simulink model "ThreephaseInverterTrialOut"  (R2016a)
settings: Solver=FixedStepAuto  StartTime=0  StopTime=time  FixedStep=Ts1  RelTol=1  AbsTol=0.1
undefined symbols (not defined in the file or in its folder): f, Ts, Ts1, Vs, Vt
libraries: nesl_utility x12, elec_lib x7, fl_lib x6, pe_lib x6, powerlib_meascontrol x1, powerlib x1
settings Model: Creator=syf  LastModifiedBy=syf

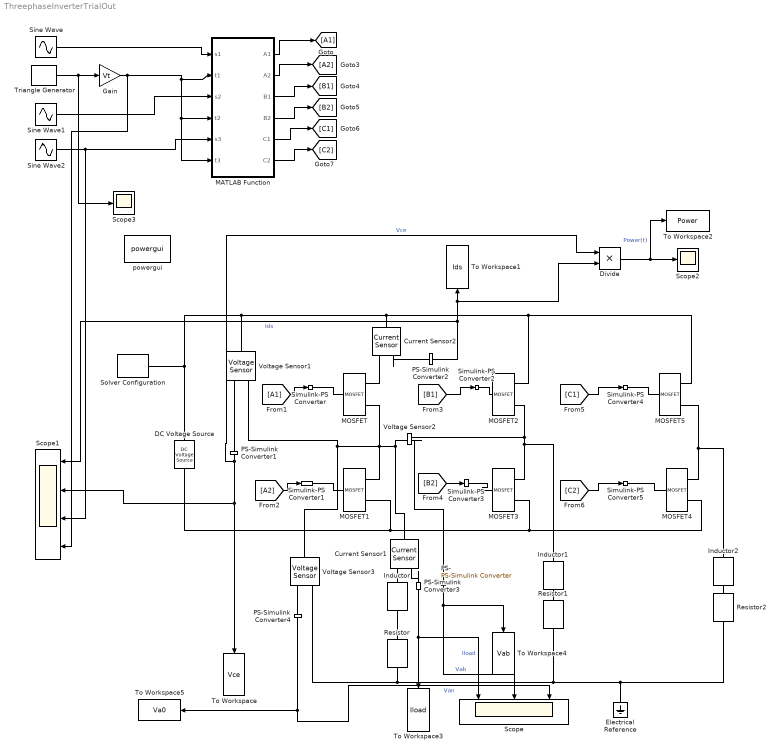
== system ThreephaseInverterTrialOut ==
  Current Sensor1 : fl_lib/Electrical/Electrical Sensors/Current Sensor
  Current Sensor2 : fl_lib/Electrical/Electrical Sensors/Current Sensor
  DC Voltage Source : elec_lib/Additional Components/SPICE-Compatible Components/Sources/DC Voltage Source  DC=650 V
  Divide : Product  Inputs=**
  Electrical Reference : fl_lib/Electrical/Electrical Elements/Electrical Reference
  Gain : Gain  Gain=Vt
  Inductor : elec_lib/Passive Devices/Inductor  l=Ls H  L_tol=20  enable_L_tol=0  tol_distribution=1  nSigma=4  r=0 Ohm  g=1e-9 1/Ohm  initI=0 A  enable_operating_limits=0  operating_limit_action=2  max_working_current=1 A  power_rating=1 W  enable_faults=0  fault_action=1  lambdaPercent=50  k_faulted=0.9999 Ohm  turnsShort=0  openCct=0  groundShort=0  groundShortG=0 1/Ohm  tau_fault=0.001 s  enable_temporal_fault=0  t_fault=1 s  enable_behavioral_fault=0  max_permissible_voltage=100 V  n_fail_on_voltage=1  max_permissible_current=1 A  t_fail_on_current=1 s
  Inductor1 : elec_lib/Passive Devices/Inductor  l=Ls H  L_tol=20  enable_L_tol=0  tol_distribution=1  nSigma=4  r=0 Ohm  g=1e-9 1/Ohm  initI=0 A  enable_operating_limits=0  operating_limit_action=2  max_working_current=1 A  power_rating=1 W  enable_faults=0  fault_action=1  lambdaPercent=50  k_faulted=0.9999 Ohm  turnsShort=0  openCct=0  groundShort=0  groundShortG=0 1/Ohm  tau_fault=0.001 s  enable_temporal_fault=0  t_fault=1 s  enable_behavioral_fault=0  max_permissible_voltage=100 V  n_fail_on_voltage=1  max_permissible_current=1 A  t_fail_on_current=1 s
  Inductor2 : elec_lib/Passive Devices/Inductor  l=Ls H  L_tol=20  enable_L_tol=0  tol_distribution=1  nSigma=4  r=0 Ohm  g=1e-9 1/Ohm  initI=0 A  enable_operating_limits=0  operating_limit_action=2  max_working_current=1 A  power_rating=1 W  enable_faults=0  fault_action=1  lambdaPercent=50  k_faulted=0.9999 Ohm  turnsShort=0  openCct=0  groundShort=0  groundShortG=0 1/Ohm  tau_fault=0.001 s  enable_temporal_fault=0  t_fault=1 s  enable_behavioral_fault=0  max_permissible_voltage=100 V  n_fail_on_voltage=1  max_permissible_current=1 A  t_fail_on_current=1 s
  MATLAB Function : MATLAB Function  TreatAsAtomicUnit=on
  MOSFET{,1..5} (6 alike) : pe_lib/Semiconductors/Fundamental Components/MOSFET  Rds=0.01 Ohm  Goff=1e-6 1/Ohm  Vth=2 V  diode_param=2  diode_Vf=0.8 V  diode_Ron=0.001 Ohm  diode_Goff=1e-5 1/Ohm  diode_C=5e-8 F  diode_iRM=-235 A  diode_iF=300 A  diode_idot=-50 A/us  diode_trr_param=1  diode_trr_factor=3  diode_trr=15 us  diode_Qrr=1.5e+3 s*uA
  "PS- " : nesl_utility/PS-Simulink Converter  PhysicalDomain=network_engine_domain  SubClassName=ps_output  LeftPortType=input  RightPortType=output  PseudoPeriodic=off  Frequencies=[]  Unit=1  AffineConversion=off
  PS-Simulink Converter{1..4} (4 alike) : nesl_utility/PS-Simulink Converter  PhysicalDomain=network_engine_domain  SubClassName=ps_output  LeftPortType=input  RightPortType=output  PseudoPeriodic=off  Frequencies=[]  Unit=1  AffineConversion=off
  Resistor : elec_lib/Passive Devices/Resistor  R=20 Ohm  R_tol=5  enable_R_tol=0  tol_distribution=1  nSigma=4  enable_operating_limits=0  operating_limit_action=2  max_working_voltage=100 V  power_rating=1 W  enable_faults=0  fault_action=1  R_faulted=Inf Ohm  enable_temporal_fault=0  t_fault=1 s  enable_behavioral_fault=0  max_permissible_current=1 A  t_fail_on_current=1 s  noise_mode=0  sample_time=0.001 s  repeatability=1  auto_seed=2843309574  user_seed=0  Tdevice=25 degC  alpha=0.00393 1/K  Tmeas=25 degC  thermal_mass=100 J/K  initial_temperature=25 degC  power_derating_T1=70 degC  power_derating_T2=155 degC  operating_temperature_range_vec=[ -50 150 ] degC
  Resistor1 : elec_lib/Passive Devices/Resistor  R=20 Ohm  R_tol=5  enable_R_tol=0  tol_distribution=1  nSigma=4  enable_operating_limits=0  operating_limit_action=2  max_working_voltage=100 V  power_rating=1 W  enable_faults=0  fault_action=1  R_faulted=Inf Ohm  enable_temporal_fault=0  t_fault=1 s  enable_behavioral_fault=0  max_permissible_current=1 A  t_fail_on_current=1 s  noise_mode=0  sample_time=0.001 s  repeatability=1  auto_seed=1846498393  user_seed=0  Tdevice=25 degC  alpha=0.00393 1/K  Tmeas=25 degC  thermal_mass=100 J/K  initial_temperature=25 degC  power_derating_T1=70 degC  power_derating_T2=155 degC  operating_temperature_range_vec=[ -50 150 ] degC
  Resistor2 : elec_lib/Passive Devices/Resistor  R=20 Ohm  R_tol=5  enable_R_tol=0  tol_distribution=1  nSigma=4  enable_operating_limits=0  operating_limit_action=2  max_working_voltage=100 V  power_rating=1 W  enable_faults=0  fault_action=1  R_faulted=Inf Ohm  enable_temporal_fault=0  t_fault=1 s  enable_behavioral_fault=0  max_permissible_current=1 A  t_fail_on_current=1 s  noise_mode=0  sample_time=0.001 s  repeatability=1  auto_seed=3812947214  user_seed=0  Tdevice=25 degC  alpha=0.00393 1/K  Tmeas=25 degC  thermal_mass=100 J/K  initial_temperature=25 degC  power_derating_T1=70 degC  power_derating_T2=155 degC  operating_temperature_range_vec=[ -50 150 ] degC
  Scope : Scope  NumInputPorts=3
  Scope1 : Scope  NumInputPorts=4
  Scope2 : Scope
  Scope3 : Scope
  Simulink-PS Converter{,1..5} (6 alike) : nesl_utility/Simulink-PS Converter  PhysicalDomain=network_engine_domain  SubClassName=ps_input  LeftPortType=input  RightPortType=output  PseudoPeriodic=off  Frequencies=[]  NoiseDistribution=none  NoiseParameters=[]  Unit=1  AffineConversion=off  InputFiltering=off  SimscapeFilterOrder=1  InputFilterTimeConstant=0.001  UdotUserProvided=1
  Sine Wave : Sin  Amplitude=Vs  Frequency=f*2*pi  SampleTime=0
  Sine Wave1 : Sin  Amplitude=Vs  Frequency=f*2*pi  Phase=2/3*pi  SampleTime=0
  Sine Wave2 : Sin  Amplitude=Vs  Frequency=f*2*pi  Phase=-2/3*pi  SampleTime=0
  Solver Configuration : nesl_utility/Solver Configuration  PhysicalDomain=network_engine_domain  SubClassName=solver  LeftPortType=input  RightPortType=generic  Accelerate=off  Tones=[]  Harmonics=[]  SimulateNoise=off  Profile=off  UseLocalSampling=off  EnableSwitchedLinearOptims=on  FrequencyDomain=off  UseCCode=off  RelTol=0.001  AbsTol=1e-06  MinStep=1e-09  ToWorkspace=off  RevertToSquareIcSolve=off  NumHomotopyIterations=100  PhasorMode=off  PhasorModeNumHarmonics=1  OverrideAbsTol=off  DoDC=off  ResidualTolerance=1e-9  UseLocalSolver=off  LocalSolverChoice=NE_BACKWARD_EULER_ADVANCER  LocalSolverSampleTime=0.001  DoFixedCost=off  MaxNonlinIter=3  MaxModeIter=2  LinearAlgebra=Sparse  DelaysMemoryBudget=1024  AutomaticFiltering=on  FilteringTimeConstant=0.001
  To Workspace : ToWorkspace  VariableName=Vce  SaveFormat=Structure With Time  SampleTime=-1
      settings: Save2DSignal=2-D array (concatenate along first dimension)
  To Workspace1 : ToWorkspace  VariableName=Ids  SaveFormat=Structure With Time  SampleTime=-1
  To Workspace2 : ToWorkspace  VariableName=Power  SampleTime=-1
  To Workspace3 : ToWorkspace  VariableName=Iload  SaveFormat=Structure With Time  SampleTime=-1
      settings: Save2DSignal=2-D array (concatenate along first dimension)
  To Workspace4 : ToWorkspace  VariableName=Vab  SaveFormat=Structure With Time  SampleTime=-1
      settings: Save2DSignal=2-D array (concatenate along first dimension)
  To Workspace5 : ToWorkspace  VariableName=Va0  SaveFormat=Structure With Time  SampleTime=-1
      settings: Save2DSignal=2-D array (concatenate along first dimension)
  Triangle Generator : powerlib_meascontrol/Pulse & Signal Generators/Triangle Generator  Freq=f_sw  Phase=90  Ts=Ts1
  Voltage Sensor1 : fl_lib/Electrical/Electrical Sensors/Voltage Sensor
  Voltage Sensor2 : fl_lib/Electrical/Electrical Sensors/Voltage Sensor
  Voltage Sensor3 : fl_lib/Electrical/Electrical Sensors/Voltage Sensor
  powergui : powerlib/powergui  Priority=1  SimulationMode=Discrete  SolverType=Tustin/Backward Euler (TBE)  SampleTime=Ts  frequency=60  SPID=off  DisableSnubberDevices=off  DisableRonSwitches=off  DisableVfSwitches=off  SwTol=0  DisplayEquations=off  Interpol=off  ExternalGateDelay=off  methode=off  Ts=10  FunctionMessages=off  echomessages=off  HookPort=off  EnableUseOfTLC=off  x0status=blocks  frequencyindice=60  Pbase=100e6  ErrMax=1e-4  Iterations=50  UnitsV=kV  UnitsW=MW  buscounter=0  RestoreLinks=warning  ResistiveCurrentMeasurement=off  Frange=[0:2:500]  Ylog=off  Xlog=on  ShowGrid=off  save=off  variable=ZData  structure=Vce  ZoomFFT=off  StartTime=0.0  cycles=1  DisplayStyle=1  fundamental=50  FreqAxis=off  MaxFrequency=10000  frequencyindicesteady=1  RmsSteady=1  display=off
  wires:
  Triangle Generator/1 -> Scope3/1, Gain/1
  Sine Wave/1 -> MATLAB Function/1(s1)
  Gain/1 -> Scope1/4, MATLAB Function/2(t1), MATLAB Function/6(t3), MATLAB Function/4(t2)
  MATLAB Function/1(A1) -> [A1]
  Sine Wave1/1 -> MATLAB Function/3(s2)
  Sine Wave2/1 -> Scope1/3, MATLAB Function/5(s3)
  MATLAB Function/2(A2) -> [A2]
  MATLAB Function/3(B1) -> [B1]
  MATLAB Function/4(B2) -> [B2]
  MATLAB Function/5(C1) -> [C1]
  MATLAB Function/6(C2) -> [C2]
  [A1] -> Simulink-PS Converter/1
  [A2] -> Simulink-PS Converter1/1
  [B1] -> Simulink-PS Converter2/1
  [B2] -> Simulink-PS Converter3/1
  [C1] -> Simulink-PS Converter4/1
  [C2] -> Simulink-PS Converter5/1
  "PS- "/1 -> To Workspace4/1, Scope/2  "Vab"
  PS-Simulink Converter3/1 -> Scope/1, To Workspace3/1  "Iload"
  PS-Simulink Converter1/1 -> To Workspace/1, Scope1/2, Divide/1  "Vce"
  PS-Simulink Converter2/1 -> Divide/2, To Workspace1/1, Scope1/1  "Ids"
  Divide/1 -> To Workspace2/1, Scope2/1  "Power(t)"
  PS-Simulink Converter4/1 -> Scope/3, To Workspace5/1  "Van"
  connections:
  Inductor/RConn1 -- Resistor/LConn1
  MOSFET2/RConn2 -- Inductor1/LConn1 -- MOSFET3/RConn1 -- Voltage Sensor2/RConn2
  Inductor2/RConn1 -- Resistor2/LConn1
  Solver Configuration/RConn1 -- Current Sensor2/LConn1 -- MOSFET2/RConn1 -- MOSFET5/RConn1 -- Voltage Sensor1/LConn1 -- DC Voltage Source/LConn1
  MOSFET3/RConn2 -- MOSFET4/RConn2 -- MOSFET1/RConn2 -- DC Voltage Source/RConn1
  Simulink-PS Converter/RConn1 -- MOSFET/LConn1
  Simulink-PS Converter1/RConn1 -- MOSFET1/LConn1
  Simulink-PS Converter2/RConn1 -- MOSFET2/LConn1
  Simulink-PS Converter3/RConn1 -- MOSFET3/LConn1
  Simulink-PS Converter4/RConn1 -- MOSFET5/LConn1
  Simulink-PS Converter5/RConn1 -- MOSFET4/LConn1
  Resistor/RConn1 -- Voltage Sensor3/RConn2 -- Resistor2/RConn1 -- Electrical Reference/LConn1 -- Resistor1/RConn1
  Voltage Sensor2/RConn1 -- "PS- "/LConn1
  MOSFET/RConn2 -- Voltage Sensor1/RConn2 -- Voltage Sensor3/LConn1 -- MOSFET1/RConn1 -- Current Sensor1/LConn1 -- Voltage Sensor2/LConn1
  Inductor1/RConn1 -- Resistor1/LConn1
  Inductor2/LConn1 -- MOSFET5/RConn2 -- MOSFET4/RConn1
  Current Sensor1/RConn2 -- Inductor/LConn1
  PS-Simulink Converter3/LConn1 -- Current Sensor1/RConn1
  PS-Simulink Converter1/LConn1 -- Voltage Sensor1/RConn1
  Current Sensor2/RConn2 -- MOSFET/RConn1
  Current Sensor2/RConn1 -- PS-Simulink Converter2/LConn1
  PS-Simulink Converter4/LConn1 -- Voltage Sensor3/RConn1

== matlab function ThreephaseInverterTrialOut/MATLAB Function ==
  data: s1 input; A1 output; t1 input; A2 output; s2 input; t2 input; s3 input; t3 input; B1 output; B2 output; C1 output; C2 output
function [A1, A2, B1, B2,C1, C2] = fcn(s1,t1,s2,t2,s3,t3)
    if s1>t1 
        A1=10;
        A2=0;
    else 
        A1=0;
        A2=10;
    end
    
    if s2>t2
        B1=10;
        B2=0;
    else 
        B1=0;
        B2=10;
    end
    
    if s3>t3
        C1=10;
        C2=0;
    else 
        C1=0;
        C2=10;
    end
